simulink model "PTB_ConventionalModel"  (R2024a)
settings: Solver=ode23tb  StartTime=0.0  StopTime=150  RelTol=1e-4  AbsTol=1e-6
model workspace (MAT data in the model file):
  Af = 4
  Cd = 0.3
  D = 0.322411602927
  DownShiftSpeeds = [11.05 18.7 28.9 38.675 51.425 11.05 18.7 28.9 38.675 51.425 11.05 18.7 ... (85 elements, 5x17)]
  DrCycles : object (value not decoded)
  I = 0.25
  Kbr = 10000
  P = 15
  PedalPositions = [0 6.2485 12.4969 18.7454 24.9939 31.2424 37.4908 43.7393 49.9878 56.2363 62.4847 68.7332 ... (17 elements, 1x17)]
  TimeHWFET = 765
  TimeUDDS = 1372
  TimeUS06 = 596
  UpShiftSpeeds = [12.75 20.997635 31.45 42.16136 55.58864 12.75 20.997635 31.45 42.16136 55.58864 12.75 20.997635 ... (85 elements, 5x17)]
  axle_b = 10
  axle_k = 5000
  convAxle_wc = 500
  diffRatio = 3.4
  driveshaft_b = 10
  driveshaft_k = 2500
  driveshaft_wc = 500
  engineSpeedPoints_rpm = [750 1053.57142857 1357.14285714 1660.71428571 1964.28571429 2267.85714286 2571.42857143 2875 3178.57142857 3482.14285714 3785.71428571 4089.28571429 ... (15 elements, 1x15)]
  engineTorqueMap_Nm = [-13.6738264269 15.0034460821 26.4289521305 37.8539339756 49.2854604964 60.7146317399 72.0173711595 77.7345012802 77.7345012802 77.7345012802 77.7345012802 77.7345012802 ... (240 elements, 16x15)]
  engineTorquePoints_Nm = [0 15 26.4285714286 37.8571428571 49.2857142857 60.7142857143 72.1428571429 83.5714285714 95 106.428571429 117.857142857 129.285714286 ... (16 elements, 1x16)]
  vehicleMass = 1500
  wheelRadius = 0.35
values from neighbouring files (symbols this model uses):
  m = 0:0.01:10    [acc_GA.m]
  s = tf('s')    [PIDTune_GeneticAlgorithm.m]    (also in pidtest.m; plots_GA.m; tf_acc_deneme.m)
libraries: Wheels_Driver_VehDyn_Lib x6, autolibsharedcoupling x4, simulink x4, autolibshareddiff x2, autolibsharedtransfixedgear x2, autolibsharedmappedengines x2, autolibshared x1, slpidlib x1
(part 5 of 5)

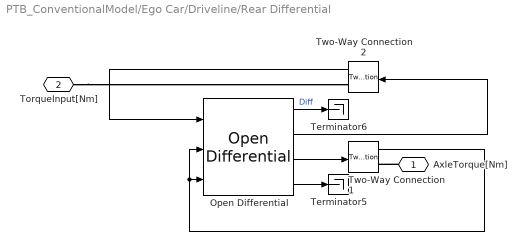
== system PTB_ConventionalModel/Ego Car/Driveline/Rear Differential ==
  Open Differential : autolibshareddiff/Open Differential  DiffEffModelPopup=Constant  InterpMethod=Linear point-slope  extTamb=off  shaftSwitchMask=To the left of center-line  Ndiff=diffRatio  Jd=.025  bd=1e-3  Jw1=.01  bw1=1e-3  Jw2=.01  bw2=1e-3  omegaw1o=0  omegaw2o=0  eta=1  eta_tbl=reshape([0.64 0.76 0.8 0.81 0.83 0.84 0.84 0.56 0.73 0.78 0.8 0.83 0.84 0.84 0.54 0.71 0.77 0.8 0.82 0.84 0.84 0.53 0.71 0.77 0.8 0.83 0.84 0.84 0.51 0.71 0.77 0.8 0.83 0.84 0.85 0.52 0.7 0.77 0.8 0.83 0.84 0.85 0.51 0.71 0.76 0.79 0.83 0.84 0.85 0.5 0.69 0.76 0.79 0.82 0.84 0.85 0.45 0.68 0.75 0.78 0.82 0.84 0.85 0.43 0.67 0.74 0.78 0.81 0.83 0.84 0.38 0.63 0.71 0.75 0.8 0.82 0.83 0.81 0.86 0.88 0.89 0.89 0.89 0.9 0.77 0.85 0.87 0.88 0.89 0.9 0.9 0.72 0.82 0.86 0.87 0.88 0.89 0.9 0.68 0.8 0.84 0.86 0.88 0.89 0.89 0.67 0.8 0.84 0.86 0.88 0.89 0.9 0.67 0.8 0.84 0.86 0.88 0.89 0.9 0.65 0.8 0.84 0.86 0.88 0.89 0.9 0.64 0.79 0.83 0.86 0.88 0.89 0.9 0.63 0.78 0.83 0.86 0.88 0.89 0.9 0.59 0.76 0.82 0.85 0.87 0.89 0.9 0.53 0.73 0.8 0.83 0.86 0.88 0.89], 7, 11, 2)  Trq_bpts=[25, 50, 75, 100, 150, 200, 250]  omega_bpts=[52.4 78.5 105 131 157 183 209 262 314 419 524]  Temp_bpts=[290 358]  Tamb=297.15  maxAbsSpd=5e3  aMode=1
      settings: LibrarySourceBlock=autolibdiff/Open Differential
  Terminator5 : Terminator
  Terminator6 : Terminator
  Two-Way Connection1 : TwoWayConnection
  Two-Way Connection2 : TwoWayConnection
  AxleTorque[Nm] : PMIOPort  Side=Right
  TorqueInput[Nm] : PMIOPort  Port=2  Side=Left
  wires:
  Open Differential/3 -> Two-Way Connection1/1
  Open Differential/4 -> Terminator5/1
  Open Differential/1 -> Terminator6/1  "Diff"
  Open Differential/2 -> Two-Way Connection2/1
  Two-Way Connection1/1 -> Open Differential/2, Open Differential/3
  Two-Way Connection2/1 -> Open Differential/1
  connections:
  AxleTorque[Nm]/RConn1 -- Two-Way Connection1/RConn1
  TorqueInput[Nm]/RConn1 -- Two-Way Connection2/RConn1

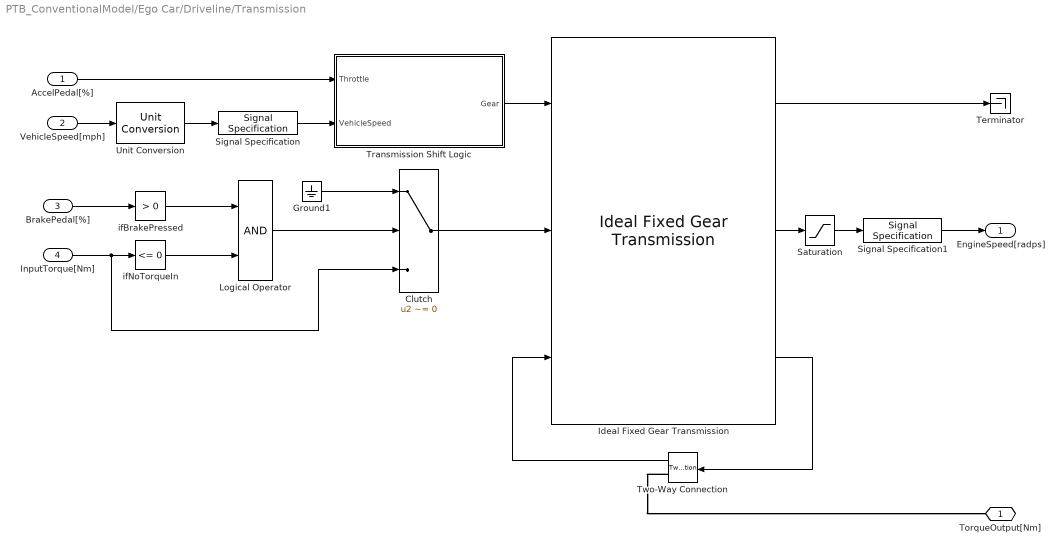
== system PTB_ConventionalModel/Ego Car/Driveline/Transmission ==
  AccelPedal[%] : Inport
  VehicleSpeed[mph] : Inport  Port=2
  BrakePedal[%] : Inport  Port=3
  InputTorque[Nm] : Inport  Port=4
  Clutch : Switch  Criteria=u2 ~= 0  SaturateOnIntegerOverflow=off  InputSameDT=off
  Ground1 : Ground
  Ideal Fixed Gear Transmission : autolibsharedtransfixedgear/Ideal Fixed Gear Transmission  VariantControl=0  TransEffModelPopup=Gear only  gearInterp=Linear point-slope  G=[-1, 0, 1, 2, 3, 4, 5, 6]  Trq_bpts=[25, 50, 75, 100, 150, 200, 250]  omega_bpts=[52.4 78.5 105 131 157 183 209 262 314 419 524]  Temp_bpts=[313 358]  N=[-4.47 ,4.47, 4.47, 2.47, 1.47, 1, 0.8 .65]  Jout=[0.128 0.01 0.128 0.1 0.062 0.028 0.01 .01]  bout=[.003 .001 .003 .0025 .002 .001 .001 .001]  eta=[0.9, 0.9, 0.9, 0.9, 0.9, 0.95, 0.95, 0.95]  eta_tbl=reshape([0.53 0.71 0.77 0.79 0.82 0.82 0.82 0.5 0.7 0.77 0.79 0.82 0.82 0.82 0.54 0.72 0.78 0.81 0.83 0.82 0.82 0.56 0.73 0.79 0.81 0.84 0.82 0.82 0.58 0.74 0.79 0.82 0.84 0.82 0.82 0.57 0.74 0.79 0.82 0.84 0.82 0.82 0.58 0.74 0.79 0.82 0.84 0.82 0.82 0.58 0.74 0.79 0.82 0.84 0.82 0.82 0.57 0.74 0.8 0.82 0.85 0.82 0.82 0.55 0.73 0.78 0.81 0.84 0.82 0.82 0.51 0.71 0.77 0.81 0.84 0.82 0.82 0.53 0.71 0.77 0.79 0.82 0.82 0.82 0.5 0.7 0.77 0.79 0.82 0.82 0.82 0.54 0.72 0.78 0.81 0.83 0.82 0.82 0.56 0.73 0.79 0.81 0.84 0.82 0.82 0.58 0.74 0.79 0.82 0.84 0.82 0.82 0.57 0.74 0.79 0.82 0.84 0.82 0.82 0.58 0.74 0.79 0.82 0.84 0.82 0.82 0.58 0.74 0.79 0.82 0.84 0.82 0.82 0.57 0.74 0.8 0.82 0.85 0.82 0.82 0.55 0.73 0.78 0.81 0.84 0.82 0.82 0.51 0.71 0.77 0.81 0.84 0.82 0.82 0.53 0.71 0.77 0.79 0.82 0.82 0.82 0.5 0.7 0.77 0.79 0.82 0.82 0.82 0.54 0.72 0.78 0.81 0.83 0.82 0.82 0.56 0.73 0.79 0.81 0.84 0.82 0.82 0.58 0.74 0.79 0.82 0.84 0.82 0.82 0.57 0.74 0.79 0.82 0.84 0.82 0.82 0.58 0.74 0.79 0.82 0.84 0.82 0.82 0.58 0.74 0.79 0.82 0.84 0.82 0.82 0.57 0.74 0.8 0.82 0.85 0.82 0.82 0.55 0.73 0.78 0.81 0.84 0.82 0.82 0.51 0.71 0.77 0.81 0.84 0.82 0.82 0.7 0.79 0.82 0.83 0.84 0.84 0.84 0.63 0.76 0.8 0.82 0.83 0.84 0.84 0.58 0.74 0.79 0.81 0.83 0.84 0.84 0.58 0.74 0.79 0.81 0.83 0.84 0.84 0.58 0.74 0.79 0.81 0.84 0.84 0.84 0.57 0.73 0.78 0.81 0.84 0.85 0.84 0.57 0.73 0.79 0.81 0.84 0.85 0.84 0.56 0.73 0.78 0.81 0.83 0.85 0.84 0.55 0.73 0.78 0.81 0.84 0.85 0.84 0.52 0.71 0.77 0.8 0.83 0.85 0.84 0.48 0.69 0.76 0.79 0.83 0.84 0.84 0.64 0.76 0.8 0.81 0.83 0.84 0.84 0.56 0.73 0.78 0.8 0.83 0.84 0.84 0.54 0.71 0.77 0.8 0.82 0.84 0.84 0.53 0.71 0.77 0.8 0.83 0.84 0.84 0.51 0.71 0.77 0.8 0.83 0.84 0.85 0.52 0.7 0.77 0.8 0.83 0.84 0.85 0.51 0.71 0.76 0.79 0.83 0.84 0.85 0.5 0.69 0.76 0.79 0.82 0.84 0.85 0.45 0.68 0.75 0.78 0.82 0.84 0.85 0.43 0.67 0.74 0.78 0.81 0.83 0.84 0.38 0.63 0.71 0.75 0.8 0.82 0.83 0.65 0.79 0.84 0.85 0.88 0.89 0.89 0.56 0.75 0.81 0.83 0.86 0.88 0.89 0.52 0.72 0.79 0.83 0.86 0.88 0.88 0.51 0.72 0.79 0.83 0.86 0.88 0.89 0.49 0.71 0.78 0.82 0.86 0.88 0.89 0.47 0.7 0.78 0.82 0.86 0.87 0.88 0.45 0.69 0.77 0.81 0.85 0.87 0.88 0.4 0.67 0.75 0.8 0.84 0.86 0.88 0.3 0.64 0.73 0.78 0.83 0.86 0.87 0.17 0.55 0.67 0.73 0.8 0.83 0.85 0.089 0.45 0.61 0.69 0.77 0.81 0.83 0.61 0.75 0.82 0.84 0.87 0.87 0.88 0.54 0.73 0.8 0.82 0.86 0.87 0.88 0.51 0.71 0.79 0.82 0.86 0.87 0.88 0.52 0.72 0.79 0.82 0.86 0.87 0.89 0.52 0.72 0.8 0.83 0.86 0.88 0.89 0.53 0.72 0.79 0.82 0.86 0.87 0.89 0.5 0.7 0.78 0.82 0.86 0.88 0.88 0.46 0.69 0.77 0.81 0.85 0.87 0.88 0.4 0.67 0.75 0.8 0.83 0.86 0.88 0.33 0.64 0.73 0.78 0.83 0.85 0.87 0.33 0.64 0.73 0.78 0.83 0.85 0.87 0.78 0.85 0.87 0.88 0.89 0.89 0.89 0.73 0.83 0.86 0.88 0.89 0.89 0.89 0.72 0.83 0.86 0.88 0.89 0.89 0.89 0.72 0.83 0.87 0.89 0.9 0.89 0.89 0.72 0.83 0.87 0.88 0.9 0.89 0.89 0.71 0.83 0.87 0.88 0.9 0.89 0.89 0.71 0.83 0.86 0.88 0.9 0.89 0.89 0.7 0.82 0.86 0.88 0.9 0.89 0.89 0.69 0.82 0.86 0.88 0.9 0.89 0.89 0.67 0.81 0.86 0.88 0.9 0.89 0.89 0.63 0.79 0.85 0.87 0.89 0.89 0.89 0.78 0.85 0.87 0.88 0.89 0.89 0.89 0.73 0.83 0.86 0.88 0.89 0.89 0.89 0.72 0.83 0.86 0.88 0.89 0.89 0.89 0.72 0.83 0.87 0.89 0.9 0.89 0.89 0.72 0.83 0.87 0.88 0.9 0.89 0.89 0.71 0.83 0.87 0.88 0.9 0.89 0.89 0.71 0.83 0.86 0.88 0.9 0.89 0.89 0.7 0.82 0.86 0.88 0.9 0.89 0.89 0.69 0.82 0.86 0.88 0.9 0.89 0.89 0.67 0.81 0.86 0.88 0.9 0.89 0.89 0.63 0.79 0.85 0.87 0.89 0.89 0.89 0.78 0.85 0.87 0.88 0.89 0.89 0.89 0.73 0.83 0.86 0.88 0.89 0.89 0.89 0.72 0.83 0.86 0.88 0.89 0.89 0.89 0.72 0.83 0.87 0.89 0.9 0.89 0.89 0.72 0.83 0.87 0.88 0.9 0.89 0.89 0.71 0.83 0.87 0.88 0.9 0.89 0.89 0.71 0.83 0.86 0.88 0.9 0.89 0.89 0.7 0.82 0.86 0.88 0.9 0.89 0.89 0.69 0.82 0.86 0.88 0.9 0.89 0.89 0.67 0.81 0.86 0.88 0.9 0.89 0.89 0.63 0.79 0.85 0.87 0.89 0.89 0.89 0.82 0.87 0.88 0.89 0.89 0.89 0.89 0.81 0.87 0.89 0.89 0.9 0.9 0.89 0.76 0.85 0.87 0.89 0.9 0.89 0.89 0.72 0.83 0.86 0.88 0.89 0.89 0.89 0.72 0.83 0.86 0.88 0.89 0.9 0.89 0.71 0.82 0.86 0.88 0.89 0.9 ...(+1314 chars))  G_o=0  omega_o=0  omegaN_o=0  tau_s=.01  maxAbsSpd=5e3  aMode=aMode
  Logical Operator : Logic  AllPortsSameDT=off  OutDataTypeStr=boolean
  Saturation : Saturate  UpperLimit=6000  LowerLimit=500
  Signal Specification : SignalSpecification  Unit=km/h
  Signal Specification1 : SignalSpecification  Unit=rad/s
  Terminator : Terminator
  Transmission Shift Logic : Stateflow chart  TreatAsAtomicUnit=on
  Two-Way Connection : TwoWayConnection
  Unit Conversion : UnitConversion
  ifBrakePressed : simulink/Logic and Bit Operations/Compare To Constant  relop=>  const=0  OutDataTypeStr=boolean
  ifNoTorqueIn : simulink/Logic and Bit Operations/Compare To Constant  relop=<=  const=0  OutDataTypeStr=boolean
  TorqueOutput[Nm] : PMIOPort  Side=Right
  EngineSpeed[radps] : Outport  VectorParamsAs1DForOutWhenUnconnected=off
  wires:
  Ideal Fixed Gear Transmission/1 -> Terminator/1
  Signal Specification1/1 -> EngineSpeed[radps]/1
  Transmission Shift Logic/1(Gear) -> Ideal Fixed Gear Transmission/1
  Ideal Fixed Gear Transmission/2 -> Saturation/1
  Two-Way Connection/1 -> Ideal Fixed Gear Transmission/3
  Unit Conversion/1 -> Signal Specification/1
  VehicleSpeed[mph]/1 -> Unit Conversion/1
  Signal Specification/1 -> Transmission Shift Logic/2(VehicleSpeed)
  AccelPedal[%]/1 -> Transmission Shift Logic/1(Throttle)
  Saturation/1 -> Signal Specification1/1
  Ideal Fixed Gear Transmission/3 -> Two-Way Connection/1
  Clutch/1 -> Ideal Fixed Gear Transmission/2
  BrakePedal[%]/1 -> ifBrakePressed/1
  Ground1/1 -> Clutch/1
  InputTorque[Nm]/1 -> Clutch/3, ifNoTorqueIn/1
  ifBrakePressed/1 -> Logical Operator/1
  Logical Operator/1 -> Clutch/2
  ifNoTorqueIn/1 -> Logical Operator/2
  connections:
  Two-Way Connection/RConn1 -- TorqueOutput[Nm]/RConn1

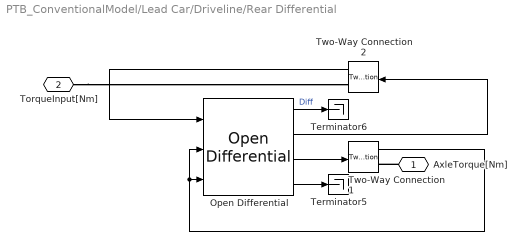
== system PTB_ConventionalModel/Lead Car/Driveline/Rear Differential ==
  Open Differential : autolibshareddiff/Open Differential  DiffEffModelPopup=Constant  InterpMethod=Linear point-slope  extTamb=off  shaftSwitchMask=To the left of center-line  Ndiff=diffRatio  Jd=.025  bd=1e-3  Jw1=.01  bw1=1e-3  Jw2=.01  bw2=1e-3  omegaw1o=0  omegaw2o=0  eta=1  eta_tbl=reshape([0.64 0.76 0.8 0.81 0.83 0.84 0.84 0.56 0.73 0.78 0.8 0.83 0.84 0.84 0.54 0.71 0.77 0.8 0.82 0.84 0.84 0.53 0.71 0.77 0.8 0.83 0.84 0.84 0.51 0.71 0.77 0.8 0.83 0.84 0.85 0.52 0.7 0.77 0.8 0.83 0.84 0.85 0.51 0.71 0.76 0.79 0.83 0.84 0.85 0.5 0.69 0.76 0.79 0.82 0.84 0.85 0.45 0.68 0.75 0.78 0.82 0.84 0.85 0.43 0.67 0.74 0.78 0.81 0.83 0.84 0.38 0.63 0.71 0.75 0.8 0.82 0.83 0.81 0.86 0.88 0.89 0.89 0.89 0.9 0.77 0.85 0.87 0.88 0.89 0.9 0.9 0.72 0.82 0.86 0.87 0.88 0.89 0.9 0.68 0.8 0.84 0.86 0.88 0.89 0.89 0.67 0.8 0.84 0.86 0.88 0.89 0.9 0.67 0.8 0.84 0.86 0.88 0.89 0.9 0.65 0.8 0.84 0.86 0.88 0.89 0.9 0.64 0.79 0.83 0.86 0.88 0.89 0.9 0.63 0.78 0.83 0.86 0.88 0.89 0.9 0.59 0.76 0.82 0.85 0.87 0.89 0.9 0.53 0.73 0.8 0.83 0.86 0.88 0.89], 7, 11, 2)  Trq_bpts=[25, 50, 75, 100, 150, 200, 250]  omega_bpts=[52.4 78.5 105 131 157 183 209 262 314 419 524]  Temp_bpts=[290 358]  Tamb=297.15  maxAbsSpd=5e3  aMode=1
      settings: LibrarySourceBlock=autolibdiff/Open Differential
  Terminator5 : Terminator
  Terminator6 : Terminator
  Two-Way Connection1 : TwoWayConnection
  Two-Way Connection2 : TwoWayConnection
  AxleTorque[Nm] : PMIOPort  Side=Right
  TorqueInput[Nm] : PMIOPort  Port=2  Side=Left
  wires:
  Open Differential/3 -> Two-Way Connection1/1
  Open Differential/4 -> Terminator5/1
  Open Differential/1 -> Terminator6/1  "Diff"
  Open Differential/2 -> Two-Way Connection2/1
  Two-Way Connection1/1 -> Open Differential/2, Open Differential/3
  Two-Way Connection2/1 -> Open Differential/1
  connections:
  AxleTorque[Nm]/RConn1 -- Two-Way Connection1/RConn1
  TorqueInput[Nm]/RConn1 -- Two-Way Connection2/RConn1

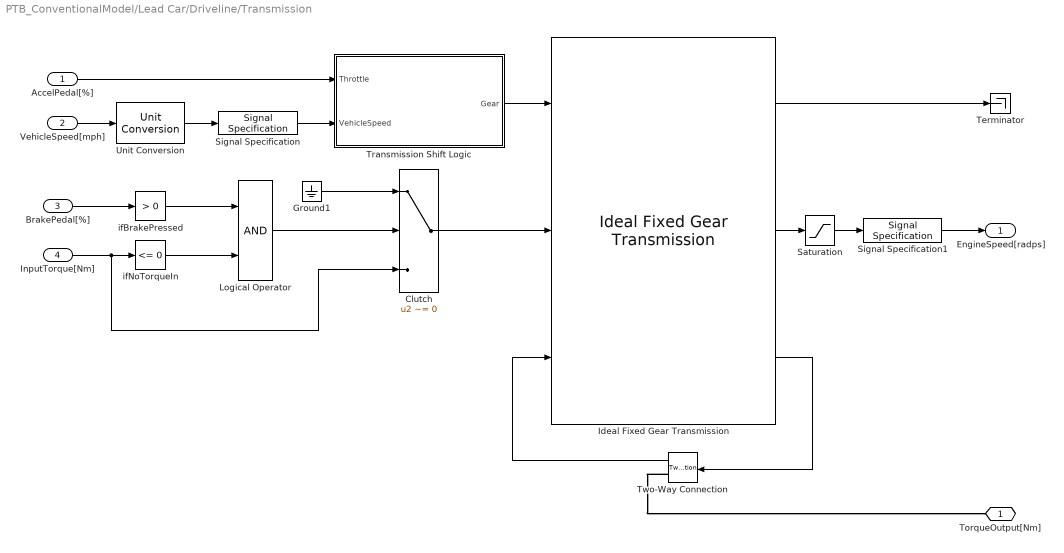
== system PTB_ConventionalModel/Lead Car/Driveline/Transmission ==
  AccelPedal[%] : Inport
  VehicleSpeed[mph] : Inport  Port=2
  BrakePedal[%] : Inport  Port=3
  InputTorque[Nm] : Inport  Port=4
  Clutch : Switch  Criteria=u2 ~= 0  SaturateOnIntegerOverflow=off  InputSameDT=off
  Ground1 : Ground
  Ideal Fixed Gear Transmission : autolibsharedtransfixedgear/Ideal Fixed Gear Transmission  VariantControl=0  TransEffModelPopup=Gear only  gearInterp=Linear point-slope  G=[-1, 0, 1, 2, 3, 4, 5, 6]  Trq_bpts=[25, 50, 75, 100, 150, 200, 250]  omega_bpts=[52.4 78.5 105 131 157 183 209 262 314 419 524]  Temp_bpts=[313 358]  N=[-4.47 ,4.47, 4.47, 2.47, 1.47, 1, 0.8 .65]  Jout=[0.128 0.01 0.128 0.1 0.062 0.028 0.01 .01]  bout=[.003 .001 .003 .0025 .002 .001 .001 .001]  eta=[0.9, 0.9, 0.9, 0.9, 0.9, 0.95, 0.95, 0.95]  eta_tbl=reshape([0.53 0.71 0.77 0.79 0.82 0.82 0.82 0.5 0.7 0.77 0.79 0.82 0.82 0.82 0.54 0.72 0.78 0.81 0.83 0.82 0.82 0.56 0.73 0.79 0.81 0.84 0.82 0.82 0.58 0.74 0.79 0.82 0.84 0.82 0.82 0.57 0.74 0.79 0.82 0.84 0.82 0.82 0.58 0.74 0.79 0.82 0.84 0.82 0.82 0.58 0.74 0.79 0.82 0.84 0.82 0.82 0.57 0.74 0.8 0.82 0.85 0.82 0.82 0.55 0.73 0.78 0.81 0.84 0.82 0.82 0.51 0.71 0.77 0.81 0.84 0.82 0.82 0.53 0.71 0.77 0.79 0.82 0.82 0.82 0.5 0.7 0.77 0.79 0.82 0.82 0.82 0.54 0.72 0.78 0.81 0.83 0.82 0.82 0.56 0.73 0.79 0.81 0.84 0.82 0.82 0.58 0.74 0.79 0.82 0.84 0.82 0.82 0.57 0.74 0.79 0.82 0.84 0.82 0.82 0.58 0.74 0.79 0.82 0.84 0.82 0.82 0.58 0.74 0.79 0.82 0.84 0.82 0.82 0.57 0.74 0.8 0.82 0.85 0.82 0.82 0.55 0.73 0.78 0.81 0.84 0.82 0.82 0.51 0.71 0.77 0.81 0.84 0.82 0.82 0.53 0.71 0.77 0.79 0.82 0.82 0.82 0.5 0.7 0.77 0.79 0.82 0.82 0.82 0.54 0.72 0.78 0.81 0.83 0.82 0.82 0.56 0.73 0.79 0.81 0.84 0.82 0.82 0.58 0.74 0.79 0.82 0.84 0.82 0.82 0.57 0.74 0.79 0.82 0.84 0.82 0.82 0.58 0.74 0.79 0.82 0.84 0.82 0.82 0.58 0.74 0.79 0.82 0.84 0.82 0.82 0.57 0.74 0.8 0.82 0.85 0.82 0.82 0.55 0.73 0.78 0.81 0.84 0.82 0.82 0.51 0.71 0.77 0.81 0.84 0.82 0.82 0.7 0.79 0.82 0.83 0.84 0.84 0.84 0.63 0.76 0.8 0.82 0.83 0.84 0.84 0.58 0.74 0.79 0.81 0.83 0.84 0.84 0.58 0.74 0.79 0.81 0.83 0.84 0.84 0.58 0.74 0.79 0.81 0.84 0.84 0.84 0.57 0.73 0.78 0.81 0.84 0.85 0.84 0.57 0.73 0.79 0.81 0.84 0.85 0.84 0.56 0.73 0.78 0.81 0.83 0.85 0.84 0.55 0.73 0.78 0.81 0.84 0.85 0.84 0.52 0.71 0.77 0.8 0.83 0.85 0.84 0.48 0.69 0.76 0.79 0.83 0.84 0.84 0.64 0.76 0.8 0.81 0.83 0.84 0.84 0.56 0.73 0.78 0.8 0.83 0.84 0.84 0.54 0.71 0.77 0.8 0.82 0.84 0.84 0.53 0.71 0.77 0.8 0.83 0.84 0.84 0.51 0.71 0.77 0.8 0.83 0.84 0.85 0.52 0.7 0.77 0.8 0.83 0.84 0.85 0.51 0.71 0.76 0.79 0.83 0.84 0.85 0.5 0.69 0.76 0.79 0.82 0.84 0.85 0.45 0.68 0.75 0.78 0.82 0.84 0.85 0.43 0.67 0.74 0.78 0.81 0.83 0.84 0.38 0.63 0.71 0.75 0.8 0.82 0.83 0.65 0.79 0.84 0.85 0.88 0.89 0.89 0.56 0.75 0.81 0.83 0.86 0.88 0.89 0.52 0.72 0.79 0.83 0.86 0.88 0.88 0.51 0.72 0.79 0.83 0.86 0.88 0.89 0.49 0.71 0.78 0.82 0.86 0.88 0.89 0.47 0.7 0.78 0.82 0.86 0.87 0.88 0.45 0.69 0.77 0.81 0.85 0.87 0.88 0.4 0.67 0.75 0.8 0.84 0.86 0.88 0.3 0.64 0.73 0.78 0.83 0.86 0.87 0.17 0.55 0.67 0.73 0.8 0.83 0.85 0.089 0.45 0.61 0.69 0.77 0.81 0.83 0.61 0.75 0.82 0.84 0.87 0.87 0.88 0.54 0.73 0.8 0.82 0.86 0.87 0.88 0.51 0.71 0.79 0.82 0.86 0.87 0.88 0.52 0.72 0.79 0.82 0.86 0.87 0.89 0.52 0.72 0.8 0.83 0.86 0.88 0.89 0.53 0.72 0.79 0.82 0.86 0.87 0.89 0.5 0.7 0.78 0.82 0.86 0.88 0.88 0.46 0.69 0.77 0.81 0.85 0.87 0.88 0.4 0.67 0.75 0.8 0.83 0.86 0.88 0.33 0.64 0.73 0.78 0.83 0.85 0.87 0.33 0.64 0.73 0.78 0.83 0.85 0.87 0.78 0.85 0.87 0.88 0.89 0.89 0.89 0.73 0.83 0.86 0.88 0.89 0.89 0.89 0.72 0.83 0.86 0.88 0.89 0.89 0.89 0.72 0.83 0.87 0.89 0.9 0.89 0.89 0.72 0.83 0.87 0.88 0.9 0.89 0.89 0.71 0.83 0.87 0.88 0.9 0.89 0.89 0.71 0.83 0.86 0.88 0.9 0.89 0.89 0.7 0.82 0.86 0.88 0.9 0.89 0.89 0.69 0.82 0.86 0.88 0.9 0.89 0.89 0.67 0.81 0.86 0.88 0.9 0.89 0.89 0.63 0.79 0.85 0.87 0.89 0.89 0.89 0.78 0.85 0.87 0.88 0.89 0.89 0.89 0.73 0.83 0.86 0.88 0.89 0.89 0.89 0.72 0.83 0.86 0.88 0.89 0.89 0.89 0.72 0.83 0.87 0.89 0.9 0.89 0.89 0.72 0.83 0.87 0.88 0.9 0.89 0.89 0.71 0.83 0.87 0.88 0.9 0.89 0.89 0.71 0.83 0.86 0.88 0.9 0.89 0.89 0.7 0.82 0.86 0.88 0.9 0.89 0.89 0.69 0.82 0.86 0.88 0.9 0.89 0.89 0.67 0.81 0.86 0.88 0.9 0.89 0.89 0.63 0.79 0.85 0.87 0.89 0.89 0.89 0.78 0.85 0.87 0.88 0.89 0.89 0.89 0.73 0.83 0.86 0.88 0.89 0.89 0.89 0.72 0.83 0.86 0.88 0.89 0.89 0.89 0.72 0.83 0.87 0.89 0.9 0.89 0.89 0.72 0.83 0.87 0.88 0.9 0.89 0.89 0.71 0.83 0.87 0.88 0.9 0.89 0.89 0.71 0.83 0.86 0.88 0.9 0.89 0.89 0.7 0.82 0.86 0.88 0.9 0.89 0.89 0.69 0.82 0.86 0.88 0.9 0.89 0.89 0.67 0.81 0.86 0.88 0.9 0.89 0.89 0.63 0.79 0.85 0.87 0.89 0.89 0.89 0.82 0.87 0.88 0.89 0.89 0.89 0.89 0.81 0.87 0.89 0.89 0.9 0.9 0.89 0.76 0.85 0.87 0.89 0.9 0.89 0.89 0.72 0.83 0.86 0.88 0.89 0.89 0.89 0.72 0.83 0.86 0.88 0.89 0.9 0.89 0.71 0.82 0.86 0.88 0.89 0.9 ...(+1314 chars))  G_o=0  omega_o=0  omegaN_o=0  tau_s=.01  maxAbsSpd=5e3  aMode=aMode
  Logical Operator : Logic  AllPortsSameDT=off  OutDataTypeStr=boolean
  Saturation : Saturate  UpperLimit=6000  LowerLimit=500
  Signal Specification : SignalSpecification  Unit=km/h
  Signal Specification1 : SignalSpecification  Unit=rad/s
  Terminator : Terminator
  Transmission Shift Logic : Stateflow chart  TreatAsAtomicUnit=on
  Two-Way Connection : TwoWayConnection
  Unit Conversion : UnitConversion
  ifBrakePressed : simulink/Logic and Bit Operations/Compare To Constant  relop=>  const=0  OutDataTypeStr=boolean
  ifNoTorqueIn : simulink/Logic and Bit Operations/Compare To Constant  relop=<=  const=0  OutDataTypeStr=boolean
  TorqueOutput[Nm] : PMIOPort  Side=Right
  EngineSpeed[radps] : Outport  VectorParamsAs1DForOutWhenUnconnected=off
  wires:
  Ideal Fixed Gear Transmission/1 -> Terminator/1
  Signal Specification1/1 -> EngineSpeed[radps]/1
  Transmission Shift Logic/1(Gear) -> Ideal Fixed Gear Transmission/1
  Ideal Fixed Gear Transmission/2 -> Saturation/1
  Two-Way Connection/1 -> Ideal Fixed Gear Transmission/3
  Unit Conversion/1 -> Signal Specification/1
  VehicleSpeed[mph]/1 -> Unit Conversion/1
  Signal Specification/1 -> Transmission Shift Logic/2(VehicleSpeed)
  AccelPedal[%]/1 -> Transmission Shift Logic/1(Throttle)
  Saturation/1 -> Signal Specification1/1
  Ideal Fixed Gear Transmission/3 -> Two-Way Connection/1
  Clutch/1 -> Ideal Fixed Gear Transmission/2
  BrakePedal[%]/1 -> ifBrakePressed/1
  Ground1/1 -> Clutch/1
  InputTorque[Nm]/1 -> Clutch/3, ifNoTorqueIn/1
  ifBrakePressed/1 -> Logical Operator/1
  Logical Operator/1 -> Clutch/2
  ifNoTorqueIn/1 -> Logical Operator/2
  connections:
  Two-Way Connection/RConn1 -- TorqueOutput[Nm]/RConn1

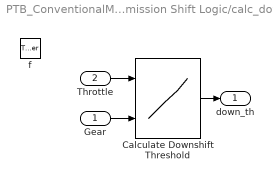
== system PTB_ConventionalModel/Ego Car/Driveline/Transmission/Transmission Shift Logic/calc_down ==
  Gear : Inport
  Throttle : Inport  Port=2
  f : TriggerPort  TriggerType=function-call  VariantControl=Variant
      settings: CopyFcn=Stateflow.SLINSF.SimulinkMan.removeBlockPreDeleteFcn  PreDeleteFcn=Stateflow.SLINSF.SimulinkMan.unsafePredeleteFcn
  Calculate Downshift Threshold : Lookup2D  RowIndex=PedalPositions  ColumnIndex=[2,3,4,5,6]  Table=DownShiftSpeeds'  LookUpMeth=Interpolation-Use End Values  SaturateOnIntegerOverflow=off  InputSameDT=off
  down_th : Outport  VectorParamsAs1DForOutWhenUnconnected=off
  wires:
  Calculate Downshift Threshold/1 -> down_th/1
  Gear/1 -> Calculate Downshift Threshold/2
  Throttle/1 -> Calculate Downshift Threshold/1

== system PTB_ConventionalModel/Ego Car/Driveline/Transmission/Transmission Shift Logic/calc_up ==
  Gear : Inport
  Throttle : Inport  Port=2
  f : TriggerPort  TriggerType=function-call  VariantControl=Variant
      settings: CopyFcn=Stateflow.SLINSF.SimulinkMan.removeBlockPreDeleteFcn  PreDeleteFcn=Stateflow.SLINSF.SimulinkMan.unsafePredeleteFcn
  Calculate Upshift Threshold : Lookup2D  RowIndex=PedalPositions  ColumnIndex=[1,2,3,4,5]  Table=UpShiftSpeeds'  LookUpMeth=Interpolation-Use End Values  SaturateOnIntegerOverflow=off  InputSameDT=off
  up_th : Outport  VectorParamsAs1DForOutWhenUnconnected=off
  wires:
  Calculate Upshift Threshold/1 -> up_th/1
  Throttle/1 -> Calculate Upshift Threshold/1
  Gear/1 -> Calculate Upshift Threshold/2

== system PTB_ConventionalModel/Lead Car/Driveline/Transmission/Transmission Shift Logic/calc_down ==
  Gear : Inport
  Throttle : Inport  Port=2
  f : TriggerPort  TriggerType=function-call  VariantControl=Variant
      settings: CopyFcn=Stateflow.SLINSF.SimulinkMan.removeBlockPreDeleteFcn  PreDeleteFcn=Stateflow.SLINSF.SimulinkMan.unsafePredeleteFcn
  Calculate Downshift Threshold : Lookup2D  RowIndex=PedalPositions  ColumnIndex=[2,3,4,5,6]  Table=DownShiftSpeeds'  LookUpMeth=Interpolation-Use End Values  SaturateOnIntegerOverflow=off  InputSameDT=off
  down_th : Outport  VectorParamsAs1DForOutWhenUnconnected=off
  wires:
  Calculate Downshift Threshold/1 -> down_th/1
  Gear/1 -> Calculate Downshift Threshold/2
  Throttle/1 -> Calculate Downshift Threshold/1

== system PTB_ConventionalModel/Lead Car/Driveline/Transmission/Transmission Shift Logic/calc_up ==
  Gear : Inport
  Throttle : Inport  Port=2
  f : TriggerPort  TriggerType=function-call  VariantControl=Variant
      settings: CopyFcn=Stateflow.SLINSF.SimulinkMan.removeBlockPreDeleteFcn  PreDeleteFcn=Stateflow.SLINSF.SimulinkMan.unsafePredeleteFcn
  Calculate Upshift Threshold : Lookup2D  RowIndex=PedalPositions  ColumnIndex=[1,2,3,4,5]  Table=UpShiftSpeeds'  LookUpMeth=Interpolation-Use End Values  SaturateOnIntegerOverflow=off  InputSameDT=off
  up_th : Outport  VectorParamsAs1DForOutWhenUnconnected=off
  wires:
  Calculate Upshift Threshold/1 -> up_th/1
  Throttle/1 -> Calculate Upshift Threshold/1
  Gear/1 -> Calculate Upshift Threshold/2

== stateflow chart PTB_ConventionalModel/Ego Car/Driveline/Transmission/Transmission Shift Logic ==
  settings: updateMethod=DISCRETE  sampleTime=0.04
  state gear_state [parallel]
    settings: executionOrder=1
    state first
      entry:
      Gear = 1;
    state second
      entry:
      Gear = 2;
    state third
      entry:
      Gear = 3;
    state fourth
      entry:
      Gear = 4;
    state fifth
      entry:
      Gear = 5;
    state sixth
      entry:
      Gear = 6;
    (default) -> first
    second -> third [order 1] : UP
    first -> second : UP
    fourth -> fifth [order 1] : UP
    fifth -> sixth [order 1] : UP
    third -> fourth [order 1] : UP
    third -> second [order 2] : DOWN
    second -> first [order 2] : DOWN
    fifth -> fourth [order 2] : DOWN
    fourth -> third [order 2] : DOWN
    sixth -> fifth : DOWN
  state selection_state [parallel]
    du:[up_th]=calc_up(Gear,Throttle);
    du:[down_th]=calc_down(Gear,Throttle);
    settings: executionOrder=2
    state steady_state
    state upshifting
    state downshifting
    (default) -> steady_state
    steady_state -> upshifting [order 1] : [VehicleSpeed > up_th]
    steady_state -> downshifting [order 2] : [VehicleSpeed < down_th && Gear > 1]
    downshifting -> steady_state [order 2] : [VehicleSpeed > down_th]
    downshifting -> steady_state [order 1] : after(1,tick)
        | [VehicleSpeed <= down_th]
        | {gear_state.DOWN;}
    upshifting -> steady_state [order 1] : after(1,tick)
        | [VehicleSpeed >= up_th]
        | {gear_state.UP;}
    upshifting -> steady_state [order 2] : [VehicleSpeed < up_th]
  state up_th = calc_up(Gear,Throttle) [function]
  state down_th = calc_down(Gear,Throttle) [function]
  data: Gear function_input; Throttle function_input; up_th function_output; Gear function_input; Throttle function_input; down_th function_output; Throttle input double [0..100]; VehicleSpeed input double; Gear output double; down_th local double; up_th local double
  events: DOWN local EITHER_EDGE_EVENT; UP local EITHER_EDGE_EVENT

== stateflow chart PTB_ConventionalModel/Lead Car/Driveline/Transmission/Transmission Shift Logic ==
  settings: updateMethod=DISCRETE  sampleTime=0.04
  state gear_state [parallel]
    settings: executionOrder=1
    state first
      entry:
      Gear = 1;
    state second
      entry:
      Gear = 2;
    state third
      entry:
      Gear = 3;
    state fourth
      entry:
      Gear = 4;
    state fifth
      entry:
      Gear = 5;
    state sixth
      entry:
      Gear = 6;
    (default) -> first
    second -> third [order 1] : UP
    first -> second : UP
    fourth -> fifth [order 1] : UP
    fifth -> sixth [order 1] : UP
    third -> fourth [order 1] : UP
    third -> second [order 2] : DOWN
    second -> first [order 2] : DOWN
    fifth -> fourth [order 2] : DOWN
    fourth -> third [order 2] : DOWN
    sixth -> fifth : DOWN
  state selection_state [parallel]
    du:[up_th]=calc_up(Gear,Throttle);
    du:[down_th]=calc_down(Gear,Throttle);
    settings: executionOrder=2
    state steady_state
    state upshifting
    state downshifting
    (default) -> steady_state
    steady_state -> upshifting [order 1] : [VehicleSpeed > up_th]
    steady_state -> downshifting [order 2] : [VehicleSpeed < down_th && Gear > 1]
    downshifting -> steady_state [order 2] : [VehicleSpeed > down_th]
    downshifting -> steady_state [order 1] : after(1,tick)
        | [VehicleSpeed <= down_th]
        | {gear_state.DOWN;}
    upshifting -> steady_state [order 1] : after(1,tick)
        | [VehicleSpeed >= up_th]
        | {gear_state.UP;}
    upshifting -> steady_state [order 2] : [VehicleSpeed < up_th]
  state up_th = calc_up(Gear,Throttle) [function]
  state down_th = calc_down(Gear,Throttle) [function]
  data: Gear function_input; Throttle function_input; up_th function_output; Gear function_input; Throttle function_input; down_th function_output; Throttle input double [0..100]; VehicleSpeed input double; Gear output double; down_th local double; up_th local double
  events: DOWN local EITHER_EDGE_EVENT; UP local EITHER_EDGE_EVENT
